simulink model "stateMachineTest"  (R2021b)
settings: Solver=FixedStepDiscrete  StartTime=0.0  StopTime=10.0  FixedStep=1e-3  RelTol=1e-3
undefined symbols (not defined in the file): sigbuilder_block
settings Model: Creator=ACH  LastModifiedBy=ACH

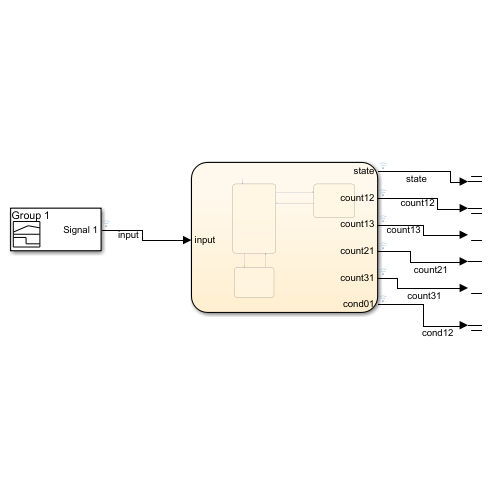
[thumbnail: Simulink's stored preview of the top-level diagram]
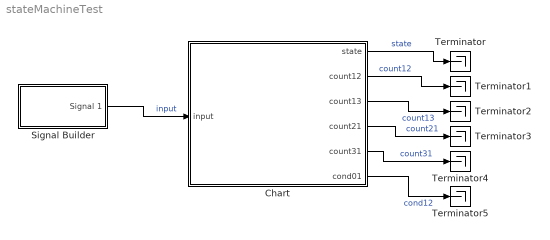
== system stateMachineTest ==
  Chart : Stateflow chart  TreatAsAtomicUnit=on
  Signal Builder : Subsystem  Tag=STV Subsys  LoadFcn=sigbuilder_block('load');  StartFcn=sigbuilder_block('start');  StopFcn=sigbuilder_block('stop');  ClipboardFcn=sigbuilder_block('clipboard');  mask(Sigbuilder block){tuvar=[0:10]}
      mask help: Simulink:masks:SigbuilderBlock_MD
      mask init:
      | if ~strcmp(get_param(bdroot(gcbh),'SimulationStatus'),'stopped') tuvar = sigbuilder_block('maskInit'); end
      settings: CopyFcn=sigbuilder_block('copy');  DeleteFcn=sigbuilder_block('delete');  ModelCloseFcn=sigbuilder_block('modelClose');  PreSaveFcn=sigbuilder_block('preSave');  PauseFcn=sigbuilder_block('pause');  ContinueFcn=sigbuilder_block('continue');  NameChangeFcn=sigbuilder_block('namechange');  OpenFcn=sigbuilder_block('open',[6 30 1428 681.75 ]);  CloseFcn=sigbuilder_block('close');
      mask Display: plot(0, 0, 100, 100,[2, 2, 32, 32, 2], [68, 8, 8, 68, 68],[32, 2], [38, 38], [32, 19, 2],[53, 60, 44], [32, 17, 17, 2],[16, 16, 31, 31]);txt = getActiveGroup(gcbh);text(2, 100, txt,'verticalAlignment', 'top');
  Terminator{,1..5} (6 alike) : Terminator
  wires:
  Signal Builder/1(Signal 1) -> Chart/1(input)  "input"
  Chart/1(state) -> Terminator/1  "state"
  Chart/2(count12) -> Terminator1/1  "count12"
  Chart/3(count13) -> Terminator2/1  "count13"
  Chart/4(count21) -> Terminator3/1  "count21"
  Chart/5(count31) -> Terminator4/1  "count31"
  Chart/6(cond01) -> Terminator5/1  "cond12"

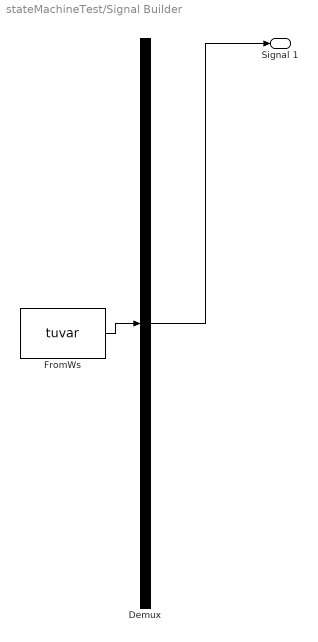
== system stateMachineTest/Signal Builder ==
  Demux : Demux  Tag=STV Demux  Outputs=1
      settings: DisplayOption=none
  FromWs : FromWorkspace  Tag=STV FromWs  VariableName=tuvar
      SigBuilderData=|
      | common.afterFinalStr = 'Extrapolate'
      | common.sampleTime = 0
      | dataSet.timeRange = [0 10]
      | dataSet.name = 'Group 1'
      | sbobj.Groups.Name = 'Group 1'
      | sbobj.Groups.Signals.Name = 'Signal 1'
      | sbobj.Groups.Signals.XData = [0 2 2 3 3 5 5 6.01 6.01 10]
      | sbobj.Groups.Signals.YData = [0 0 1 1 0 0 2 2 0 0]
  Signal 1 : Outport  Tag=STV Outport
  wires:
  Demux/1 -> Signal 1/1
  FromWs/1 -> Demux/1

== stateflow chart stateMachineTest/Chart ==
  state FIRST
    %on after(2,sec):
    state = 0;
    input1 = input;
    entry:
    count12 = 0;
    count13 = 0;
    during:
    if (input == 1)
    count12 = count12 + 1;
    else
    count12 = 0;
    end
    cond01 = (input==1);
    if (input==2)
    count13 = count13 + 1;
    else
    count13 = 0;
    end
    exit:
    count12 = 0;
    count13 = 0;
  state SECOND
    %on after(2,sec):
    state = 1;
    entry: count21 = 0;
    during:
    if (input==0)
    count21 = count21 + 1;
    else
    count21 = 0;
    end
    exit: count21 = 0;
  state THIRD
    %on after(2,sec):
    state = 2;
    entry: count31 = 0;
    during:
    if (input==0)
    count31 = count31 + 1;
    else
    count31 = 0;
    end
    exit: count31 = 0;
  (default) -> FIRST
  FIRST -> SECOND [order 2] : [(input==1)&(count12==51)]
  SECOND -> FIRST : [(input == 0)&(count21==51)]
  FIRST -> THIRD [order 1] : [(input == 2)&(count13==51)]
  THIRD -> FIRST : [(input == 0)&(count31==51)]
  data: input input; state output; count12 output; count13 output; count21 output; count31 output; input1 local; cond01 output
